simulink model "ekf2lct"  (R2014a)
settings: Solver=FixedStepDiscrete  StartTime=0.0  StopTime=100.0  RelTol=1e-3
values from neighbouring files (symbols this model uses):
  T = block.DialogPrm(6).Data    [sfall2.m]    (also in sysall.m = 0.05)
undefined symbols (not defined in the file or in its folder): phi_0, psi_0, Q, R, theta_0, V_0
libraries: simulink x3
settings Model: Creator=gcampa  LastModifiedBy=gcampa
settings DataIOCC: SignalLoggingSaveFormat=ModelDataLogs  SaveOutput=off  SignalLogging=off  DSMLogging=off  SaveTime=off
settings OptimizationCC: ExpressionDepthLimit=2147483647  InitFltsAndDblsToZero=on
settings DebuggingCC: SaveWithParameterizedLinksMsg=none  UnderspecifiedInitializationDetection=Classic  SignalResolutionControl=TryResolveAllWithWarning  MultiTaskDSMMsg=warning  MultiTaskCondExecSysMsg=none  FcnCallInpInsideContextMsg=UseLocalSettings  StateNameClashWarn=warning  StrictBusMsg=None
settings SFSimCC: SimParseCustomCode=off
settings RTWCC: IncludeERTFirstTime=on  RTWCompilerOptimization=On
settings GRTTargetCC: TargetFcnLib=ansi_tfl_tmw.mat  CombineOutputUpdateFcns=off  GRTInterface=on

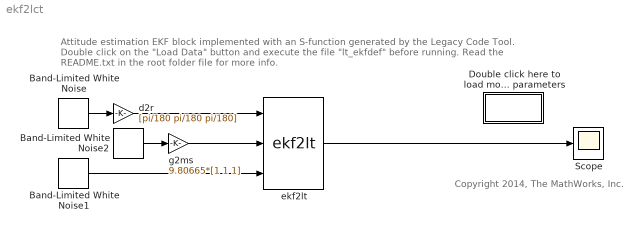
== system ekf2lct ==
  note: Copyright 2014, The MathWorks, Inc.
  note: Attitude estimation EKF block implemented with an S-function generated by the Legacy Code Tool.
      | Double click on the "Load Data" button and execute the file "lt_ekfdef" before running.
      | Read the README.txt in the root folder file for more info.
  Band-Limited White Noise : simulink/Sources/Band-Limited White Noise  Cov=0.1*[1 1 1]  Ts=T  seed=[1 2 3]
  Band-Limited White Noise1 : simulink/Sources/Band-Limited White Noise  Cov=0.1*[1 1 1]  Ts=T  seed=[7 8 9]
  Band-Limited White Noise2 : simulink/Sources/Band-Limited White Noise  Cov=0.1*[1 1 1]  Ts=T  seed=[4 5 6]
  Double click here to load model and parameters : Subsystem
      settings: OpenFcn=|
      | V_0= 21.44176640107837;
      | phi_0=0.16673723163960;
      | theta_0=0.38249284705297;
      | psi_0=-3.10672050096899;
      | 
      | Q= [1.1339e-006     0               0
      |     0               3.1232e-006     0
      |     0               0               2.9009e-006];
      | 
      | R= [0.3368          0               0
      |     0               0.092           0
      |     0               0               0];
      | 
      | T=0.05;
      mask Display: disp('Load\nData')
  Scope : Scope
      settings: TimeRange=100  YMin=-4  YMax=4
  d2r : Gain  Gain=[pi/180 pi/180 pi/180]  SaturateOnIntegerOverflow=on  OutDataTypeStr=Inherit: Same as input  ParamDataTypeStr=Inherit: Same as input
  ekf2lt : S-Function  FunctionName=ekf2lt  Parameters=Q(1:2,1:2),R(1:2,1:2),1e-5,T,zeros(2),[phi_0 theta_0]',[V_0*cos(psi_0) V_0*sin(psi_0) V_0*sin(theta_0)]  EnableBusSupport=off
  g2ms : Gain  Gain=9.80665*[1 1 1]  SaturateOnIntegerOverflow=on  OutDataTypeStr=Inherit: Same as input  ParamDataTypeStr=Inherit: Same as input
  wires:
  Band-Limited White Noise/1 -> d2r/1
  Band-Limited White Noise1/1 -> ekf2lt/3
  Band-Limited White Noise2/1 -> g2ms/1
  d2r/1 -> ekf2lt/1
  g2ms/1 -> ekf2lt/2
  ekf2lt/1 -> Scope/1

== system ekf2lct/Double click here to load model and parameters ==
